simulink model "eModel"  (Simulink 9.1)
settings: Solver=FixedStepAuto  StartTime=0.0  StopTime=simtime  FixedStep=0.1  RelTol=1e-3
libraries: slident x1
settings Model: Creator=Administrator  LastModifiedBy=Administrator
settings DataIOCC: SaveFormat=Dataset
settings OptimizationCC: LifeSpan=auto
settings DebuggingCC: UnderspecifiedInitializationDetection=Simplified  MergeDetectMultiDrivingBlocksExec=error  SFUnexpectedBacktrackingDiag=error  SFNoUnconditionalDefaultTransitionDiag=error  SFExecutionAtInitializationDiag=warning
settings HardwareCC: ProdBitPerPointer=64  ProdBitPerSizeT=64  ProdBitPerPtrDiffT=64  ProdLargestAtomicFloat=Float  ProdIntDivRoundTo=Zero  ProdEndianess=LittleEndian  ProdWordSize=64  ProdHWDeviceType=Intel->x86-64 (Windows64)
settings ModelReferenceCC: PropagateSignalLabelsOutOfModel=on
settings CodeAppCC: StateflowObjectComments=off
settings GRTTargetCC: TargetLangStandard=C99 (ISO)  CombineOutputUpdateFcns=on  GRTInterface=off
settings ConfigComp: CovMetricSettings=dwe  CovHtmlReporting=off  CovSaveCumulativeToWorkspaceVar=off  CovSaveSingleToWorkspaceVar=off  CovExternalEMLEnable=on

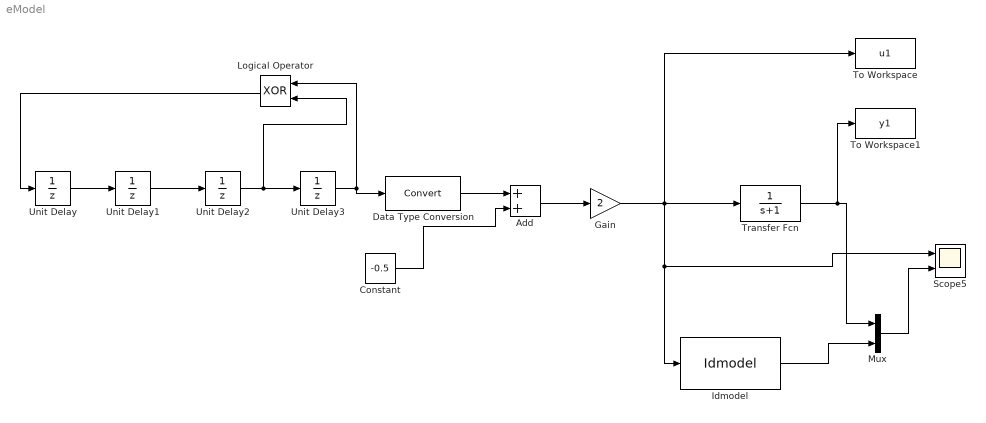
== system eModel ==
  Add : Sum
  Constant : Constant  Value=-0.5
  Data Type Conversion : DataTypeConversion
  Gain : Gain  Gain=2
  Idmodel : slident/Models/Idmodel  sys=m_est  IC=0  noi=on  seed=[]
      settings: SourceProductName=System Identification Toolbox  SourceProductBaseCode=ID
  Logical Operator : Logic  Operator=XOR  AllPortsSameDT=off  OutDataTypeStr=boolean
  Mux : Mux  Inputs=2
  Scope5 : Scope  NumInputPorts=2
  To Workspace : ToWorkspace  VariableName=u1  SampleTime=-1
  To Workspace1 : ToWorkspace  VariableName=y1  SampleTime=-1
  Transfer Fcn : TransferFcn  Denominator=[1 1]
  Unit Delay : UnitDelay  InitialCondition=1  SampleTime=-1
  Unit Delay1 : UnitDelay  SampleTime=-1
  Unit Delay2 : UnitDelay  SampleTime=-1
  Unit Delay3 : UnitDelay  SampleTime=-1
  wires:
  Logical Operator/1 -> Unit Delay/1
  Unit Delay3/1 -> Logical Operator/1, Data Type Conversion/1
  Unit Delay1/1 -> Unit Delay2/1
  Constant/1 -> Add/2
  Gain/1 -> Transfer Fcn/1, To Workspace/1, Scope5/1, Idmodel/1
  Transfer Fcn/1 -> To Workspace1/1, Mux/1
  Add/1 -> Gain/1
  Data Type Conversion/1 -> Add/1
  Unit Delay2/1 -> Logical Operator/2, Unit Delay3/1
  Unit Delay/1 -> Unit Delay1/1
  Idmodel/1 -> Mux/2
  Mux/1 -> Scope5/2
